simulink model "Calc"  (R2021a)
settings: Solver=FixedStepDiscrete  StartTime=0.0  StopTime=12  FixedStep=3  RelTol=1e-3  EnableMultiTasking=on
settings Model: Creator=alyma  LastModifiedBy=alyma
settings DataIOCC: ReturnWorkspaceOutputs=off
settings OptimizationCC: DefaultParameterBehavior=Inlined  InlineInvariantSignals=on  EnableMemcpy=off  LifeSpan=1  EfficientTunableParamExpr=on
settings DebuggingCC: UnderspecifiedInitializationDetection=Classic  MergeDetectMultiDrivingBlocksExec=none  SFMachineParentedDataDiag=warning  ArithmeticOperatorsInVariantConditions=warning
settings ModelReferenceCC: PropagateSignalLabelsOutOfModel=off
settings SFSimCC: MATLABDynamicMemAlloc=off  CustomCodeUndefinedFunction=UseInterfaceOnly
settings RTWCC: SystemTargetFile=ert.tlc  GenCodeOnly=on  TemplateMakefile=ert_default_tmf  GenerateReport=on  IncludeHyperlinkInReport=on  LaunchReport=on  GenerateTraceInfo=on  GenerateTraceReport=on  GenerateTraceReportSl=on  GenerateTraceReportSf=on  GenerateTraceReportEml=on
settings CodeAppCC: ForceParamTrailComments=on  IgnoreCustomStorageClasses=off  OperatorAnnotations=on  SimulinkDataObjDesc=on  SFDataObjDesc=on  MATLABFcnDesc=on  InsertBlockDesc=on  StateflowObjectComments=on  MATLABSourceComments=on
settings ERTTargetCC: MultiwordLength=2048  GenerateSampleERTMain=on  InlinedParameterPlacement=NonHierarchical  ERTCustomFileTemplate=example_file_process.tlc

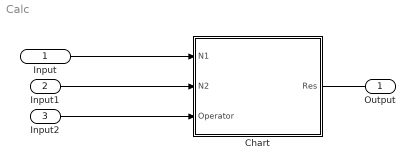
== system Calc ==
  Input : Inport
  Input1 : Inport  Port=2
  Input2 : Inport  Port=3
  Chart : Stateflow chart  TreatAsAtomicUnit=on
  Output : Outport
  wires:
  Input/1 -> Chart/1(N1)
  Chart/1(Res) -> ?
  Input1/1 -> Chart/2(N2)
  Input2/1 -> Chart/3(Operator)

== stateflow chart Calc/Chart ==
  state Add(Num1,Num2) [function]
    (default) -> (junction 2) : {Res=Num1+Num2;}
  state Calculator
    (default) -> (junction 55) : % Calc
    (junction 55) -> (junction 56) [order 1] : [Operator == 0]
    (junction 55) -> (junction 57) [order 2]
    (junction 56) -> (junction 64) : {Add(N1,N2);}
    (junction 57) -> (junction 58) [order 1] : [Operator == 1]
    (junction 57) -> (junction 59) [order 2]
    (junction 58) -> (junction 63) : {Sub(N1,N2);}
    (junction 59) -> (junction 60) [order 1] : [Operator == 2]
    (junction 59) -> (junction 61) [order 2] : {Div(N1,N2);}
    (junction 60) -> (junction 62) : {Mul(N1,N2);}
    (junction 62) -> (junction 61)
    (junction 63) -> (junction 62)
    (junction 64) -> (junction 63)
    (junction 61) -> (junction 65)
  state Sub(Num1,Num2) [function]
    (default) -> (junction 23) : {Res=Num1-Num2;}
  state Mul(Num1,Num2) [function]
    (default) -> (junction 25) : {Res=Num1*Num2;}
  state Div(Num1,Num2) [function]
    (default) -> (junction 27)
    (junction 27) -> (junction 31) [order 1] : [Num2==0]
    (junction 27) -> (junction 29) [order 2] : {Res=Num1/Num2;}
    (junction 31) -> (junction 33) : {Res=-1;}
    (junction 33) -> (junction 29)
    (junction 29) -> (junction 38)
  (default) -> Calculator
  data: Num1 function_input; Num2 function_input; Num1 function_input; Num2 function_input; Num1 function_input; Num2 function_input; Num1 function_input; Num2 function_input; N1 input; N2 input; Operator input; Res output double
